simulink model "LOKI_autotrans_AT52"  (R2022b)
settings: Solver=ode5  StartTime=0.0  StopTime=inf  FixedStep=stepsize  RelTol=1e-3  AbsTol=1e-6
model workspace (MAT data in the model file):
  CONVERTER_DATA = [0  137.465208994  2.232; 0.1  137.065019157  2.075; 0.2  135.864449646  1.975; 0.3  135.664354728  1.846; 0.4  137.565256453  1.72; 0.5  140.366585312  1.564; 0.6  145.268910814  1.409; 0.7  152.872517717  1.254; 0.8  162.9773111  1.096; 0.81  164.27792807  1.08; 0.82  166.178829795  1.061; 0.83  167.979684062  1.043; 0.84  170.080680706  1.028; 0.85  172.781962105  1.012; 0.86  175.383196045  1.002; 0.87  179.585189333  1.002; 0.88  183.587087703  1.001; 0.89  189.890077635  0.998; 0.9  197.693779455  0.999; 0.92  215.902417037  1.001; 0.94  244.515990379  1.002]
  DOWN_TABLE = [0  5  20  35; 0  5  20  35; 0  5  25  40; 0  5  30  50; 0  30  50  80; 0  30  50  80]
  DOWN_TH_BP = [0; 5; 40; 50; 90; 100]
  EMAP = [-40  -44  -49  -53  -57  -61  -65  -70  -74  -78  -82; 215  117  85  66  44  29  10  -2  -13  -22  -32; 245  208  178  148  122  104  85  66  48  33  18; 264  260  241  219  193  167  152  133  119  96  85; 264  279  282  275  260  238  223  208  189  171  152; 267  290  293  297  290  275  260  256  234  212  193; 267  297  305  305  305  301  293  282  267  249  226; 267  301  308  312  319  323  319  316  297  279  253; 267  301  312  319  327  327  327  327  312  293  267; 267  301  312  319  327  334  334  334  319  305  275]
  Iei = 0.0219914882836
  NE_VEC = [800 1200 1600 2000 2400 2800 3200 3600 4000 4400 4800]
  TH_VEC = [0; 20; 30; 40; 50; 60; 70; 80; 90; 100]
  TWAIT = 2
  UP_TABLE = [10  30  50  1000000; 10  30  50  1000000; 15  30  50  1000000; 23  41  60  1000000; 40  70  100  1000000; 40  70  100  1000000]
  UP_TH_BP = [0; 25; 35; 50; 90; 100]
  VEHICLE_DATA = [3.23; 40; 0.02; 1; 12.0941478573; 0]
values from neighbouring files (symbols this model uses):
  actionLowerLimits = [0 0]'    [LOKI_autotrans_DDPG.m]    (also in LOKI_autotrans_DDPG_AT1.m; LOKI_autotrans_DDPG_AT2.m; LOKI_autotrans_DDPG_AT51.m; system_param_settings.mat = [0 0])
  actionUpperLimits = [100 325]'    [LOKI_autotrans_DDPG.m]    (also in LOKI_autotrans_DDPG_AT1.m; LOKI_autotrans_DDPG_AT2.m; LOKI_autotrans_DDPG_AT51.m; system_param_settings.mat = [100 325])
  specHorizon = 20.1    [LOKI_autotrans_DDPG_AT1.m]    (also in LOKI_autotrans_DDPG_AT51.m = 32.7)
  stateLowerLimits = [0 0]'    [LOKI_autotrans_DDPG.m]    (also in LOKI_autotrans_DDPG_AT1.m; LOKI_autotrans_DDPG_AT2.m; LOKI_autotrans_DDPG_AT51.m; system_param_settings.mat = [0 0])
  stateUpperLimits = [5500 125]'    [LOKI_autotrans_DDPG.m]    (also in LOKI_autotrans_DDPG_AT1.m = [5000 125]'; LOKI_autotrans_DDPG_AT2.m = [5000 125]'; LOKI_autotrans_DDPG_AT51.m = [5000 125]'; system_param_settings.mat = [5500 130])
  stepsize = 0.02    [LOKI_autotrans_DDPG_AT51.m]
  tau = 20    [LOKI_autotrans_DDPG.m]
  Tf = 30    [LOKI_autotrans_DDPG.m]    (also in LOKI_autotrans_DDPG_AT1.m; LOKI_autotrans_DDPG_AT2.m; LOKI_autotrans_DDPG_AT51.m = 35)
  vmax = 120    [LOKI_autotrans_DDPG.m]
libraries: simulink x1, rllib x1
Description:
  | Modeling an Automatic Transmission Controller
  | 
  | In this example, Simulink(R) is used to model an automotive drivetrain. Stateflow(R)
  | enhances the Simulink model with its representation of the transmission
  | control logic. Simulink provides a powerful environment for the modeling and
  | simulation of dynamic systems and processes. In many systems, though,
  | supervisory functions like changing modes or invoking new gain schedules must
  | respond to events that may occur and conditions that develop over time. As a
  | result, the environment requires a language capable of managing these multiple
  | modes and developing conditions. In the following example, Stateflow
  | demonstrates its strength in this capacity by performing the function of gear
  | selection in an automatic transmission. This function is combined with the
  | drivetrain dynamics in a natural and intuitive manner by incorporating a
  | Stateflow block in the Simulink block diagram.
settings Model: DataTypeOverride=Double  MinMaxOverflowLogging=ForceOff  FPTRunName=Active  ModifiedByFormat=The MathWorks, Inc.  Creator=The MathWorks, Inc.  LastModifiedBy=The MathWorks, Inc.
settings SolverCC: AutoScaleAbsTol=off  AlgebraicLoopSolver=TrustRegion
settings DataIOCC: SaveFormat=StructureWithTime  SaveOutput=off  DSMLogging=off  InspectSignalLogs=on  SaveTime=off  SignalLoggingName=LOKI_autotrans_AT51_logsout
settings OptimizationCC: BlockReduction=off  ExpressionDepthLimit=2147483647  InitFltsAndDblsToZero=on  LifeSpan=inf
settings DebuggingCC: SignalInfNanChecking=error  SaveWithParameterizedLinksMsg=none  CheckExecutionContextPreStartOutputMsg=on  MultiTaskCondExecSysMsg=none  SigSpecEnsureSampleTimeMsg=none  IntegerOverflowMsg=none  FcnCallInpInsideContextMsg=warning  SignalLabelMismatchMsg=error  UnconnectedInputMsg=error  UnconnectedOutputMsg=error  UnconnectedLineMsg=error  UniqueDataStoreMsg=error  BusObjectLabelMismatch=error  RootOutportRequireBusObject=error  StateNameClashWarn=warning  StrictBusMsg=ErrorOnBusTreatedAsVector  NonBusSignalsTreatedAsBus=error  SymbolicDimsDataTypeCodeGenerationDiagnostic=none  SFUnexpectedBacktrackingDiag=warning  SFNoUnconditionalDefaultTransitionDiag=warning  SFExecutionAtInitializationDiag=none  SFMachineParentedDataDiag=warning  IntegerSaturationMsg=none  ArithmeticOperatorsInVariantConditions=warning
settings HardwareCC: ProdBitPerPointer=32  ProdBitPerSizeT=32  ProdBitPerPtrDiffT=32  ProdLargestAtomicFloat=None  ProdIntDivRoundTo=Floor  ProdEndianess=Unspecified  ProdWordSize=32  ProdHWDeviceType=32-bit Generic
settings ModelReferenceCC: EnableRefExpFcnMdlSchedulingChecks=on  PropagateSignalLabelsOutOfModel=off
settings SFSimCC: SFSimEcho=off  SimUseLocalCustomCode=off  SimParseCustomCode=off  CustomCodeUndefinedFunction=UseInterfaceOnly
settings RTWCC: RTWUseLocalCustomCode=off  DLArmComputeVersion=19.05
settings CodeAppCC: StateflowObjectComments=on
settings GRTTargetCC: TargetFcnLib=ansi_tfl_tmw.mat  TargetLangStandard=C89/C90 (ANSI)  CombineOutputUpdateFcns=off  GRTInterface=on
settings ConfigComp: CovMetricSettings=dcmtr  CovHTMLOptions=-aTS=1 -bRG=1 -bTC=1 -hTR=0 -nFC=0 -scm=1 -bcm=1 -xEv=0  CovSaveCumulativeToWorkspaceVar=on  CovSaveSingleToWorkspaceVar=on  CovExternalEMLEnable=off

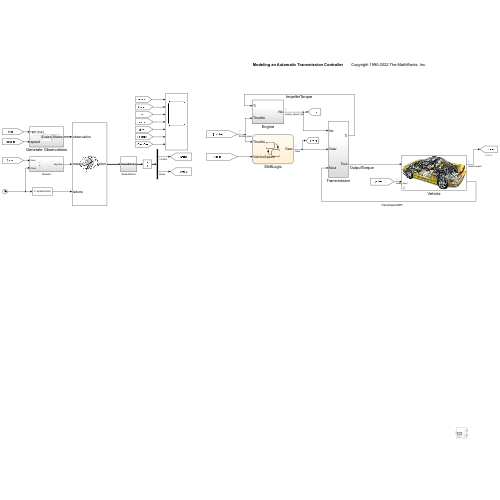
[thumbnail: Simulink's stored preview of the top-level diagram]
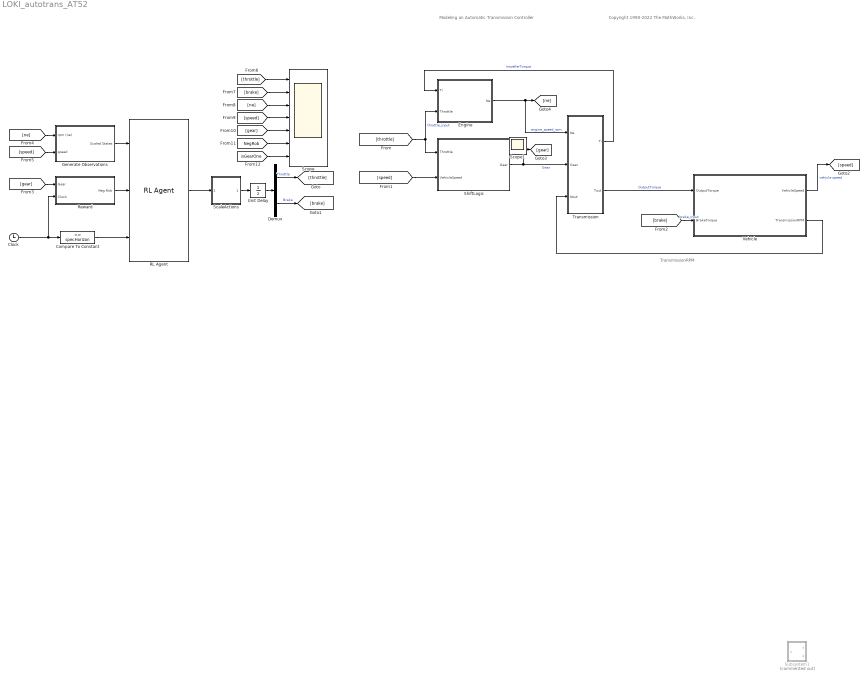
== system LOKI_autotrans_AT52 ==
  note: TransmissionRPM
  note: Modeling an Automatic Transmission Controller
  note: Copyright 1990-2022 The MathWorks, Inc.
  Clock : Clock
  Compare To Constant : simulink/Logic and Bit Operations/Compare To Constant  relop=>=  const=specHorizon  OutDataTypeStr=boolean
  Demux : Demux  Outputs=2
  Engine : Subsystem
  Generate Observations : Subsystem
  RL Agent : rllib/RL Agent  Agent=agentObj  ExternalActionAsInput=off  ProvideLastAction=off  ProvideCumRwd=off  TreatAsDirectFeedthrough=on  UseStrictObservationDataTypes=off
  Reward : Subsystem
  ScaleActions : Subsystem
  Scope : Scope  NumInputPorts=7
  ShiftLogic : Stateflow chart  TreatAsAtomicUnit=on
  Subsystem1 : Subsystem  Commented=on
  Transmission : Subsystem
  Unit Delay : UnitDelay  SampleTime=-1  HasFrameUpgradeWarning=on
  Vehicle : Subsystem  mask(vehicle model){Rfd=VEHICLE_DATA(1), rload0=VEHICLE_DATA(2), rload2=VEHICLE_DATA(3), Rw=VEHICLE_DATA(4), Iv=VEHICLE_DATA(5), N20=VEHICLE_DATA(6)/VEHICLE_DATA(4)*VEHICLE_DATA(1)}
      mask prompts: Rfd "final drive ratio"; rload0 "drag friction at wheels"; rload2 "aerodynamic drag"; Rw "wheel radius"; Iv "vehicle inertia"; N20 "initial transmission output speed"
      mask help: vehicle dynamics: torque input from trans., outputs are input speed (transmission output) and vehicle speed
      mask Display: image('$imagefile') % use "Edit Image" on toolstrip to change.
  Scope1 : Scope
  wires:
  Transmission/1(Ti) -> Engine/1(Ti)  "ImpellerTorque"
  Transmission/2(Tout) -> Vehicle/1(OutputTorque)  "OutputTorque"
  Generate Observations/1(Scaled States) -> RL Agent/1
  ShiftLogic/1(Gear) -> Transmission/2(Gear), [gear]  "Gear"
  [throttle] -> ShiftLogic/1(Throttle), Engine/2(Throttle)  "throttle_input"
  [speed] -> ShiftLogic/2(VehicleSpeed)
  [brake] -> Vehicle/2(BrakeTorque)  "brake_input"
  Clock/1 -> Reward/2(Clock), Compare To Constant/1
  RL Agent/1 -> ScaleActions/1(Raw Action from NN)
  ScaleActions/1(Rescaled Action) -> Unit Delay/1
  Demux/1 -> [throttle]  "Throttle"
  Demux/2 -> [brake]  "Brake"
  Vehicle/2(TransmissionRPM) -> Transmission/3(Nout)
  Vehicle/1(VehicleSpeed) -> [speed]  "vehicle speed"
  Compare To Constant/1 -> RL Agent/3
  Reward/1(Neg Rob) -> RL Agent/2
  [gear] -> Reward/1(Gear)
  Engine/1(Ne) -> [ne], Transmission/1(Ne)  "engine_speed_rpm"
  [ne] -> Generate Observations/1(rpm (ne))
  [speed] -> Generate Observations/2(speed)
  [throttle] -> Scope/1
  [brake] -> Scope/2
  [ne] -> Scope/3
  [speed] -> Scope/4
  [gear] -> Scope/5
  [isGearOne] -> Scope/7
  [NegRob] -> Scope/6
  Unit Delay/1 -> Demux/1

== system LOKI_autotrans_AT52/Engine ==
  note: Engine
  Ti : Inport  Unit=ft*lbf@torque
  Throttle : Inport  Port=2  Unit=%
  EnginePlusImpellerInertia : Gain  Gain=1/Iei  SaturateOnIntegerOverflow=on  OutDataTypeStr=Inherit: Same as input  ParamDataTypeStr=Inherit: Same as input
  EngineTorque : Lookup_n-D  BreakpointsForDimension1=TH_VEC  BreakpointsForDimension2=NE_VEC  Table=EMAP
      settings: InputPortMap=u0,u1
  Integrator : Integrator  InitialCondition=1000  LimitOutput=on  UpperSaturationLimit=6000  LowerSaturationLimit=600  ZeroCross=off
  Sum : Sum  Inputs=-+  InputSameDT=on  SaturateOnIntegerOverflow=on  OutDataTypeStr=Inherit: Same as first input
  Ne : Outport  Unit=rpm  VectorParamsAs1DForOutWhenUnconnected=off
  wires:
  Ti/1 -> Sum/1
  Throttle/1 -> EngineTorque/1
  Integrator/1 -> EngineTorque/2, Ne/1
  Sum/1 -> EnginePlusImpellerInertia/1
  EnginePlusImpellerInertia/1 -> Integrator/1
  EngineTorque/1 -> Sum/2

== system LOKI_autotrans_AT52/Generate Observations ==
  rpm (ne) : Inport
  speed : Inport  Port=2
  Constant : Constant  Value=-(stateLowerLimits + stateUpperLimits)./(stateUpperLimits-stateLowerLimits)
  Gain : Gain  Gain=2./(stateUpperLimits-stateLowerLimits)
  Mux1 : Mux  Inputs=2
  Sum : Sum  Inputs=|++
  Scaled States : Outport
  wires:
  speed/1 -> Mux1/2
  rpm (ne)/1 -> Mux1/1
  Mux1/1 -> Gain/1
  Sum/1 -> Scaled States/1
  Gain/1 -> Sum/1
  Constant/1 -> Sum/2

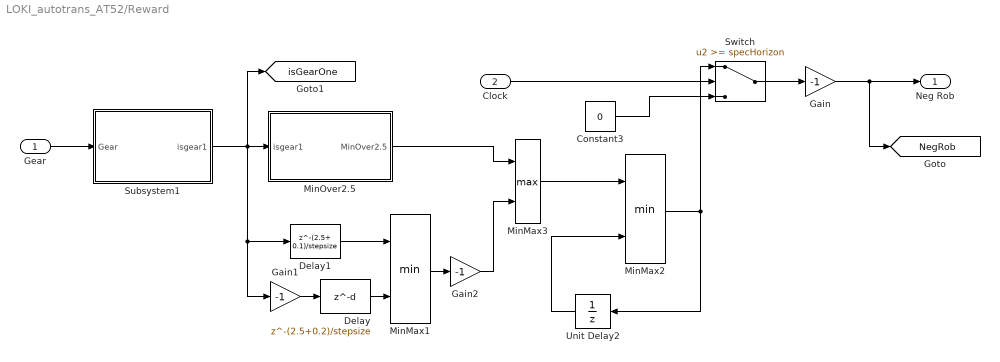
== system LOKI_autotrans_AT52/Reward ==
  Gear : Inport
  Clock : Inport  Port=2
  Constant3 : Constant  Value=0
  Delay : Delay  DelayLength=(2.5+0.2)/stepsize  InitialCondition=-1
  Delay1 : Delay  DelayLength=(2.5+ 0.1)/stepsize  InitialCondition=-1
  Gain : Gain  Gain=-1
  Gain1 : Gain  Gain=-1
  Gain2 : Gain  Gain=-1
  MinMax1 : MinMax  Inputs=2
  MinMax2 : MinMax  Inputs=2
  MinMax3 : MinMax  Function=max  Inputs=2
  MinOver2.5 : Subsystem
  Subsystem1 : Subsystem
  Switch : Switch  Threshold=specHorizon  SaturateOnIntegerOverflow=off  InputSameDT=off
  Unit Delay2 : UnitDelay  InitialCondition=10000  SampleTime=-1  HasFrameUpgradeWarning=on
  Neg Rob : Outport
  tag scope: NegRob=global, isGearOne=global
  wires:
  Constant3/1 -> Switch/3
  Switch/1 -> Gain/1
  Clock/1 -> Switch/2
  Gear/1 -> Subsystem1/1(Gear)
  Subsystem1/1(isgear1) -> [isGearOne], MinOver2.5/1(isgear1), Gain1/1, Delay1/1
  Delay/1 -> MinMax1/2
  Delay1/1 -> MinMax1/1
  MinMax2/1 -> Unit Delay2/1, Switch/1
  Gain/1 -> [NegRob], Neg Rob/1
  MinOver2.5/1(MinOver2.5) -> MinMax3/1
  Unit Delay2/1 -> MinMax2/2
  Gain1/1 -> Delay/1
  MinMax1/1 -> Gain2/1
  Gain2/1 -> MinMax3/2
  MinMax3/1 -> MinMax2/1

== system LOKI_autotrans_AT52/ScaleActions ==
  Raw Action from NN : Inport
  Constant : Constant  Value=0.5*(actionUpperLimits+actionLowerLimits)
  Gain1 : Gain  Gain=0.5*(actionUpperLimits-actionLowerLimits)
  Sum1 : Sum  Inputs=|++
  Rescaled Action : Outport
  wires:
  Gain1/1 -> Sum1/1
  Sum1/1 -> Rescaled Action/1
  Constant/1 -> Sum1/2
  Raw Action from NN/1 -> Gain1/1

== system LOKI_autotrans_AT52/ShiftLogic/ComputeThreshold ==
  note: Threshold Calculation
  Gear : Inport
  Throttle : Inport  Port=2
  f : TriggerPort  TriggerType=function-call  VariantControl=(inherit)
      settings: CopyFcn=Stateflow.SLINSF.SimulinkMan.removeBlockPreDeleteFcn  PreDeleteFcn=Stateflow.SLINSF.SimulinkMan.unsafePredeleteFcn
  InterpDown : Lookup_n-D  BreakpointsForDimension1=DOWN_TH_BP  BreakpointsForDimension2=[1:4]  Table=DOWN_TABLE  OutDataTypeStr=double  InputSameDT=off  LockScale=on
      settings: InputPortMap=u0,u1
  InterpUp : Lookup_n-D  BreakpointsForDimension1=UP_TH_BP  BreakpointsForDimension2=[1:4]  Table=UP_TABLE  OutDataTypeStr=double  InputSameDT=off  LockScale=on
      settings: InputPortMap=u0,u1
  down_th : Outport  InitialOutput=0  VectorParamsAs1DForOutWhenUnconnected=off
  up_th : Outport  Port=2  InitialOutput=0  VectorParamsAs1DForOutWhenUnconnected=off
  wires:
  InterpUp/1 -> up_th/1
  InterpDown/1 -> down_th/1
  Throttle/1 -> InterpDown/1, InterpUp/1
  Gear/1 -> InterpDown/2, InterpUp/2

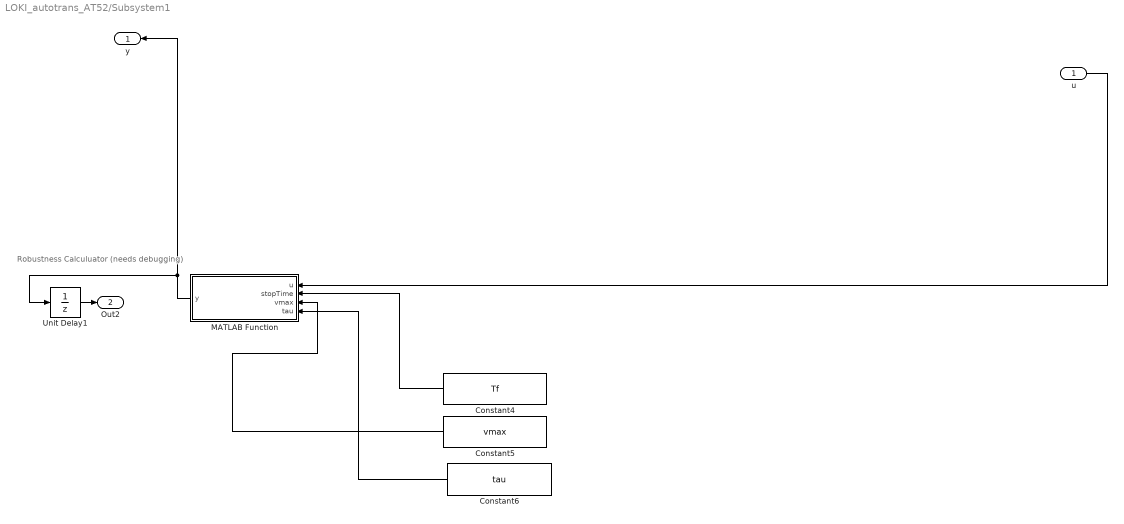
== system LOKI_autotrans_AT52/Subsystem1 ==
  note: Robustness Calculuator (needs debugging)
  u : Inport
  Constant4 : Constant  Value=Tf  VectorParams1D=off
  Constant5 : Constant  Value=vmax  VectorParams1D=off
  Constant6 : Constant  Value=tau  VectorParams1D=off
  MATLAB Function : MATLAB Function  TreatAsAtomicUnit=on
  Unit Delay1 : UnitDelay  InitialCondition=1000  SampleTime=-1  HasFrameUpgradeWarning=on
  y : Outport
  Out2 : Outport  Port=2
  wires:
  u/1 -> MATLAB Function/1(u)
  Constant4/1 -> MATLAB Function/2(stopTime)
  Constant5/1 -> MATLAB Function/3(vmax)
  MATLAB Function/1(y) -> y/1, Unit Delay1/1
  Constant6/1 -> MATLAB Function/4(tau)
  Unit Delay1/1 -> Out2/1

== system LOKI_autotrans_AT52/Transmission ==
  note: Transmission
  Ne : Inport  Unit=rpm
  Gear : Inport  Port=2  Unit=1
  Nout : Inport  Port=3  Unit=rpm
  TorqueConverter : Subsystem  mask(torque converter){speedratio=CONVERTER_DATA(:,1), Kfactor=CONVERTER_DATA(:,2), Torkratio=CONVERTER_DATA(:,3)}
      mask prompts: speedratio "speed ratio"; Kfactor "K factor"; Torkratio "torque ratio"
      mask help: torque converter
      mask Help: Torque converter input and output torques are computed as a function of the input and output speeds
      mask Display: plot([cos([90:10:450]*pi/180),.63*cos([90:10:450]*pi/180),.63*cos([90:10:240]*pi/180),cos([240:10:300]*pi/180),.63*cos([300]*pi/180)],[sin([90:10:450]*pi/180),.63*sin([90:10:450]*pi/180)+.1,.63*sin([90:10:240]*pi/180)+.1,sin([240:10:300]*pi/180),.63*sin([300]*pi/180)+.1])
  TransmissionRatio : Subsystem
  Ti : Outport  Unit=ft*lbf@torque  VectorParamsAs1DForOutWhenUnconnected=off
  Tout : Outport  Port=2  Unit=ft*lbf@torque  VectorParamsAs1DForOutWhenUnconnected=off
  wires:
  TransmissionRatio/1(Tout) -> Tout/1
  TorqueConverter/1(Ti) -> Ti/1
  Nout/1 -> TransmissionRatio/3(Nout)
  Gear/1 -> TransmissionRatio/2(Gear)
  Ne/1 -> TorqueConverter/1(Ne)
  TransmissionRatio/2(Nin) -> TorqueConverter/2(Nin)
  TorqueConverter/2(Tt) -> TransmissionRatio/1(Tin)  "TurbineTorque"

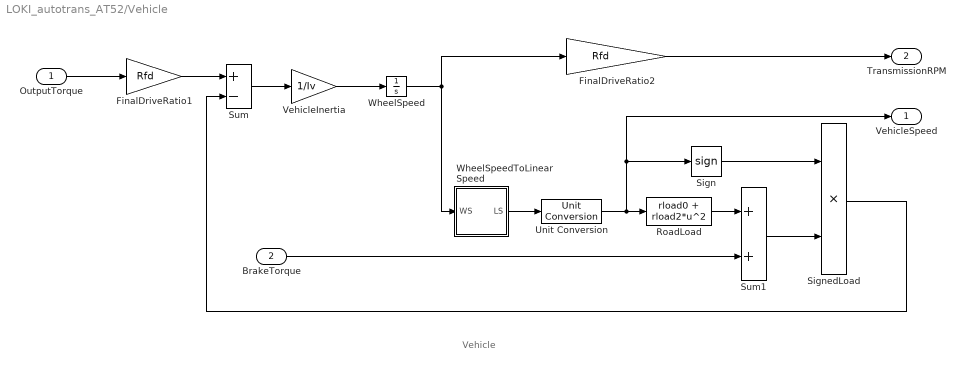
== system LOKI_autotrans_AT52/Vehicle ==
  note: Vehicle
  OutputTorque : Inport  Unit=ft*lbf@torque
  BrakeTorque : Inport  Port=2  Unit=ft*lbf@torque
  FinalDriveRatio1 : Gain  Gain=Rfd  SaturateOnIntegerOverflow=on  OutDataTypeStr=Inherit: Same as input  ParamDataTypeStr=Inherit: Same as input
  FinalDriveRatio2 : Gain  Gain=Rfd  SaturateOnIntegerOverflow=on  OutDataTypeStr=Inherit: Same as input  ParamDataTypeStr=Inherit: Same as input
  RoadLoad : Fcn  Expr=rload0 + rload2*u^2
  Sign : Signum
  SignedLoad : Product  InputSameDT=on  SaturateOnIntegerOverflow=on  OutDataTypeStr=Inherit: Same as first input
  Sum : Sum  Inputs=+-  InputSameDT=on  SaturateOnIntegerOverflow=on  OutDataTypeStr=Inherit: Same as first input
  Sum1 : Sum  InputSameDT=on  SaturateOnIntegerOverflow=on  OutDataTypeStr=Inherit: Same as first input
  Unit Conversion : UnitConversion
  VehicleInertia : Gain  Gain=1/Iv  SaturateOnIntegerOverflow=on  OutDataTypeStr=Inherit: Same as input  ParamDataTypeStr=Inherit: Same as input
  WheelSpeed : Integrator  InitialCondition=N20/Rfd  ZeroCross=off
  WheelSpeedToLinearSpeed : Subsystem
  VehicleSpeed : Outport  Unit=mph  VectorParamsAs1DForOutWhenUnconnected=off
  TransmissionRPM : Outport  Port=2  Unit=rpm  VectorParamsAs1DForOutWhenUnconnected=off
  wires:
  FinalDriveRatio2/1 -> TransmissionRPM/1
  BrakeTorque/1 -> Sum1/2
  Sum1/1 -> SignedLoad/2
  RoadLoad/1 -> Sum1/1
  Sign/1 -> SignedLoad/1
  SignedLoad/1 -> Sum/2
  OutputTorque/1 -> FinalDriveRatio1/1
  VehicleInertia/1 -> WheelSpeed/1
  Sum/1 -> VehicleInertia/1
  Unit Conversion/1 -> VehicleSpeed/1, Sign/1, RoadLoad/1
  WheelSpeed/1 -> WheelSpeedToLinearSpeed/1(WS), FinalDriveRatio2/1
  FinalDriveRatio1/1 -> Sum/1
  WheelSpeedToLinearSpeed/1(LS) -> Unit Conversion/1

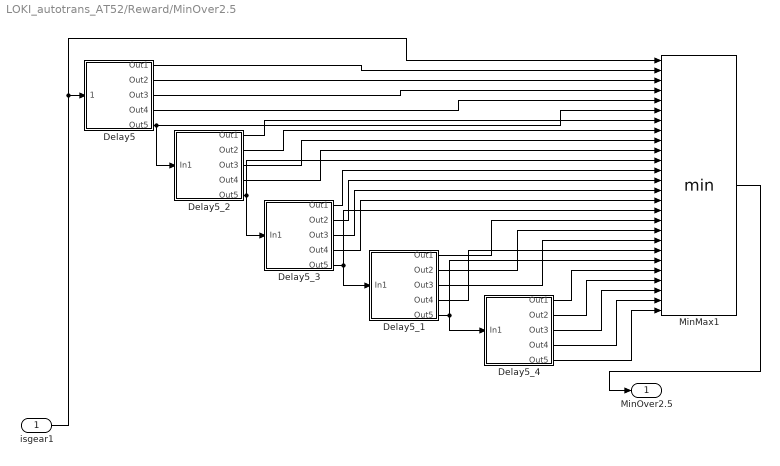
== system LOKI_autotrans_AT52/Reward/MinOver2.5 ==
  isgear1 : Inport
  Delay5 : Subsystem
  Delay5_1 : Subsystem
  Delay5_2 : Subsystem
  Delay5_3 : Subsystem
  Delay5_4 : Subsystem
  MinMax1 : MinMax  Inputs=26
  MinOver2.5 : Outport
  wires:
  Delay5_4/5(Out5) -> MinMax1/26
  Delay5_1/4(Out4) -> MinMax1/20
  Delay5_3/5(Out5) -> MinMax1/16, Delay5_1/1(In1)
  Delay5_4/1(Out1) -> MinMax1/22
  Delay5_1/5(Out5) -> Delay5_4/1(In1), MinMax1/21
  Delay5_2/5(Out5) -> MinMax1/11, Delay5_3/1(In1)
  Delay5_4/4(Out4) -> MinMax1/25
  Delay5_3/1(Out1) -> MinMax1/12
  Delay5/5(Out5) -> MinMax1/6, Delay5_2/1(In1)
  Delay5_4/2(Out2) -> MinMax1/23
  Delay5_1/3(Out3) -> MinMax1/19
  isgear1/1 -> Delay5/1(isgear1), MinMax1/1
  Delay5_1/2(Out2) -> MinMax1/18
  Delay5_3/2(Out2) -> MinMax1/13
  Delay5_1/1(Out1) -> MinMax1/17
  Delay5_2/4(Out4) -> MinMax1/10
  Delay5_4/3(Out3) -> MinMax1/24
  Delay5_3/4(Out4) -> MinMax1/15
  Delay5/1(Out1) -> MinMax1/2
  Delay5_2/3(Out3) -> MinMax1/9
  Delay5/2(Out2) -> MinMax1/3
  Delay5/4(Out4) -> MinMax1/5
  Delay5_2/1(Out1) -> MinMax1/7
  Delay5_3/3(Out3) -> MinMax1/14
  Delay5_2/2(Out2) -> MinMax1/8
  Delay5/3(Out3) -> MinMax1/4
  MinMax1/1 -> MinOver2.5/1

== system LOKI_autotrans_AT52/Reward/Subsystem1 ==
  Gear : Inport
  Add : Sum  Inputs=+-
  Add1 : Sum  Inputs=+-
  Constant : Constant  Value=0.8
  Constant1 : Constant  Value=1.2
  MinMax : MinMax  Inputs=2
  isgear1 : Outport
  wires:
  MinMax/1 -> isgear1/1  "isgear1"
  Add1/1 -> MinMax/2
  Gear/1 -> Add1/2, Add/1
  Constant/1 -> Add/2
  Add/1 -> MinMax/1
  Constant1/1 -> Add1/1

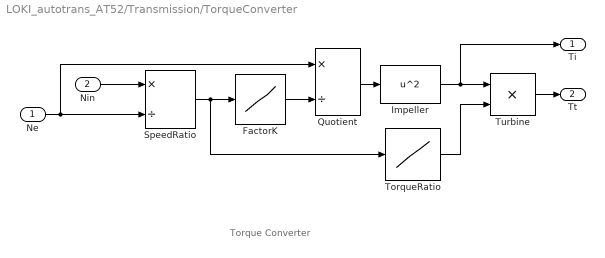
== system LOKI_autotrans_AT52/Transmission/TorqueConverter ==
  note: Torque Converter
  Ne : Inport
  Nin : Inport  Port=2
  FactorK : Lookup_n-D  NumberOfTableDimensions=1  BreakpointsForDimension1=speedratio  Table=Kfactor  SaturateOnIntegerOverflow=on
  Impeller : Fcn  Expr=u^2
  Quotient : Product  Inputs=*/  InputSameDT=on  SaturateOnIntegerOverflow=on  OutDataTypeStr=Inherit: Same as first input
  SpeedRatio : Product  Inputs=*/  InputSameDT=on  SaturateOnIntegerOverflow=on  OutDataTypeStr=Inherit: Same as first input
  TorqueRatio : Lookup_n-D  NumberOfTableDimensions=1  BreakpointsForDimension1=speedratio  Table=Torkratio  SaturateOnIntegerOverflow=on
  Turbine : Product  InputSameDT=on  SaturateOnIntegerOverflow=on  OutDataTypeStr=Inherit: Same as first input
  Ti : Outport  VectorParamsAs1DForOutWhenUnconnected=off
  Tt : Outport  Port=2  VectorParamsAs1DForOutWhenUnconnected=off
  wires:
  TorqueRatio/1 -> Turbine/2
  Quotient/1 -> Impeller/1
  FactorK/1 -> Quotient/2
  SpeedRatio/1 -> TorqueRatio/1, FactorK/1
  Impeller/1 -> Turbine/1, Ti/1
  Turbine/1 -> Tt/1
  Ne/1 -> SpeedRatio/2, Quotient/1
  Nin/1 -> SpeedRatio/1

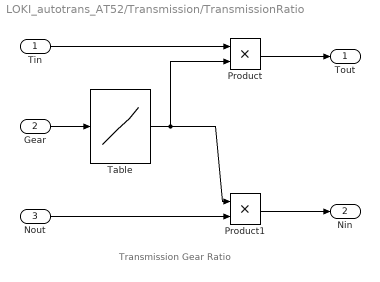
== system LOKI_autotrans_AT52/Transmission/TransmissionRatio ==
  note: Transmission Gear Ratio
  Tin : Inport  Unit=ft*lbf@torque
  Gear : Inport  Port=2  Unit=1
  Nout : Inport  Port=3  Unit=rpm
  Product : Product  InputSameDT=on  SaturateOnIntegerOverflow=on  OutDataTypeStr=Inherit: Same as first input
  Product1 : Product  InputSameDT=on  SaturateOnIntegerOverflow=on  OutDataTypeStr=Inherit: Same as first input
  Table : Lookup_n-D  NumberOfTableDimensions=1  BreakpointsForDimension1=[1 2 3 4]  Table=[2.393 1.450 1.000 0.677]  OutDataTypeStr=double  SaturateOnIntegerOverflow=on  LockScale=on
  Tout : Outport  Unit=ft*lbf@torque  VectorParamsAs1DForOutWhenUnconnected=off
  Nin : Outport  Port=2  Unit=rpm  VectorParamsAs1DForOutWhenUnconnected=off
  wires:
  Table/1 -> Product1/1, Product/2
  Nout/1 -> Product1/2
  Product1/1 -> Nin/1
  Product/1 -> Tout/1
  Tin/1 -> Product/1
  Gear/1 -> Table/1

== system LOKI_autotrans_AT52/Vehicle/WheelSpeedToLinearSpeed ==
  WS : Inport  Unit=rpm
  ToLinearSpeed : Gain  Gain=2*pi*Rw  SaturateOnIntegerOverflow=on  OutDataTypeStr=Inherit: Same as input  ParamDataTypeStr=Inherit: Same as input
  LS : Outport  Unit=ft/min  VectorParamsAs1DForOutWhenUnconnected=off
  wires:
  ToLinearSpeed/1 -> LS/1
  WS/1 -> ToLinearSpeed/1

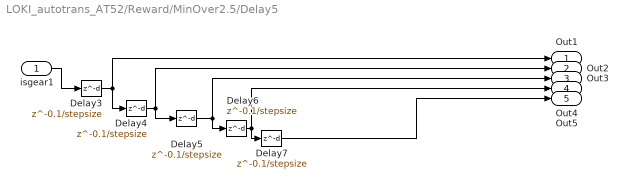
== system LOKI_autotrans_AT52/Reward/MinOver2.5/Delay5 ==
  isgear1 : Inport
  Delay{3..7} (5 alike) : Delay  DelayLength=0.1/stepsize  InitialCondition=-1
  Out1 : Outport
  Out2 : Outport  Port=2
  Out3 : Outport  Port=3
  Out4 : Outport  Port=4
  Out5 : Outport  Port=5
  wires:
  Delay4/1 -> Out2/1, Delay5/1
  isgear1/1 -> Delay3/1
  Delay6/1 -> Out4/1, Delay7/1
  Delay3/1 -> Out1/1, Delay4/1
  Delay7/1 -> Out5/1
  Delay5/1 -> Out3/1, Delay6/1

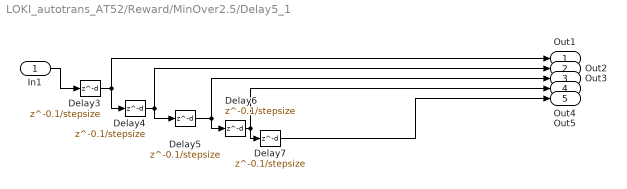
== system LOKI_autotrans_AT52/Reward/MinOver2.5/Delay5_1 ==
  In1 : Inport
  Delay{3..7} (5 alike) : Delay  DelayLength=0.1/stepsize  InitialCondition=-1
  Out1 : Outport
  Out2 : Outport  Port=2
  Out3 : Outport  Port=3
  Out4 : Outport  Port=4
  Out5 : Outport  Port=5
  wires:
  Delay5/1 -> Delay6/1, Out3/1
  Delay7/1 -> Out5/1
  Delay3/1 -> Delay4/1, Out1/1
  Delay6/1 -> Delay7/1, Out4/1
  In1/1 -> Delay3/1
  Delay4/1 -> Delay5/1, Out2/1

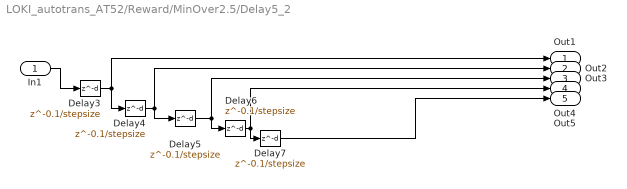
== system LOKI_autotrans_AT52/Reward/MinOver2.5/Delay5_2 ==
  In1 : Inport
  Delay{3..7} (5 alike) : Delay  DelayLength=0.1/stepsize  InitialCondition=-1
  Out1 : Outport
  Out2 : Outport  Port=2
  Out3 : Outport  Port=3
  Out4 : Outport  Port=4
  Out5 : Outport  Port=5
  wires:
  Delay5/1 -> Delay6/1, Out3/1
  Delay7/1 -> Out5/1
  Delay3/1 -> Delay4/1, Out1/1
  Delay6/1 -> Delay7/1, Out4/1
  In1/1 -> Delay3/1
  Delay4/1 -> Delay5/1, Out2/1

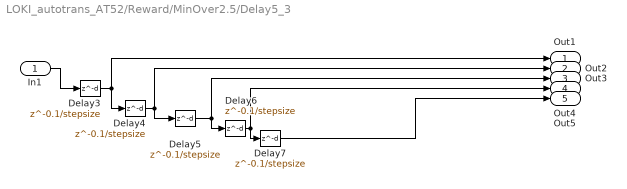
== system LOKI_autotrans_AT52/Reward/MinOver2.5/Delay5_3 ==
  In1 : Inport
  Delay{3..7} (5 alike) : Delay  DelayLength=0.1/stepsize  InitialCondition=-1
  Out1 : Outport
  Out2 : Outport  Port=2
  Out3 : Outport  Port=3
  Out4 : Outport  Port=4
  Out5 : Outport  Port=5
  wires:
  Delay4/1 -> Out2/1, Delay5/1
  In1/1 -> Delay3/1
  Delay6/1 -> Out4/1, Delay7/1
  Delay3/1 -> Out1/1, Delay4/1
  Delay7/1 -> Out5/1
  Delay5/1 -> Out3/1, Delay6/1

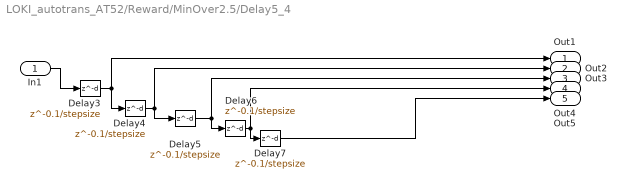
== system LOKI_autotrans_AT52/Reward/MinOver2.5/Delay5_4 ==
  In1 : Inport
  Delay{3..7} (5 alike) : Delay  DelayLength=0.1/stepsize  InitialCondition=-1
  Out1 : Outport
  Out2 : Outport  Port=2
  Out3 : Outport  Port=3
  Out4 : Outport  Port=4
  Out5 : Outport  Port=5
  wires:
  Delay4/1 -> Out2/1, Delay5/1
  In1/1 -> Delay3/1
  Delay6/1 -> Out4/1, Delay7/1
  Delay3/1 -> Out1/1, Delay4/1
  Delay7/1 -> Out5/1
  Delay5/1 -> Out3/1, Delay6/1

== stateflow chart LOKI_autotrans_AT52/ShiftLogic ==
  settings: updateMethod=DISCRETE  sampleTime=0.04
  state gear_state [parallel]
    settings: executionOrder=1
    state first
      entry:
      Gear = 1;
    state second
      entry:
      Gear = 2;
    state third
      entry:
      Gear = 3;
    state fourth
      entry:
      Gear = 4;
    (default) -> first
    second -> third [order 1] : UP
    first -> second : UP
    third -> fourth [order 1] : UP
    third -> second [order 2] : DOWN
    second -> first [order 2] : DOWN
    fourth -> third : DOWN
  state selection_state [parallel]
    during:
    [down_th, up_th] = ComputeThreshold(Gear,Throttle);
    settings: executionOrder=2
    state steady_state
    state upshifting
    state downshifting
    (default) -> steady_state
    steady_state -> upshifting [order 1] : [VehicleSpeed > up_th]
    steady_state -> downshifting [order 2] : [VehicleSpeed < down_th]
    downshifting -> steady_state [order 2] : [VehicleSpeed > down_th]
    downshifting -> steady_state [order 1] : after(TWAIT,tick)
        | [VehicleSpeed <= down_th]
        | {gear_state.DOWN}
    upshifting -> steady_state [order 1] : after(TWAIT,tick)
        | [VehicleSpeed >= up_th]
        | {gear_state.UP}
    upshifting -> steady_state [order 2] : [VehicleSpeed < up_th]
  state [down_th,up_th] = ComputeThreshold(Gear,Throttle) [function]
  data: Gear function_input; Throttle function_input; down_th function_output; up_th function_output; Throttle input double; VehicleSpeed input double; Gear output fixdt(0,8,5) [1..4]; TWAIT parameter fixdt(0,8,6); down_th local double; up_th local double
  events: DOWN local EITHER_EDGE_EVENT; UP local EITHER_EDGE_EVENT

== matlab function LOKI_autotrans_AT52/Subsystem1/MATLAB Function ==
  settings: updateMethod=DISCRETE
  data: u input; stopTime input; vmax input; tau input; y output
% u = (clock, throttle, brake, speed, rpm, gear)
function y = fcn(u,stopTime,vmax,tau)
    persistent trace  
    if(isempty(trace)) 
        trace = [];
    end
    trace = [trace u];
    if (u(1)==stopTime)
        res = 100000;
        for timeId = 1:size(trace,2)
            if (trace(1,timeId)<=tau)
                if ((vmax-trace(4,timeId)) < res)
                    res = vmax-trace(4,timeId);
                end
            end
        end        
        y = -res;
    else
        y = 0;
    end
end
